simulink model "pid_azimuth"  (Simulink 5.0)
settings: Solver=ode5  StartTime=0.0  StopTime=30  FixedStep=.01  RelTol=1e-3
undefined symbols (not defined in the file): a, b, c, control_a, force_a, rpm_a
settings Model: LastModifiedBy=Administrator

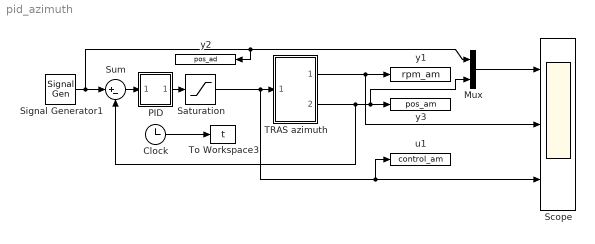
== system pid_azimuth ==
  Clock : Clock
  Mux : Mux  Inputs=2
  "PID " : Subsystem  AncestorBlock=|  mask(PID(2) Controller){P=a, I=b, D=c, N=100, S=1}
      | simulink_extras/Additional
      | Linear/PID Controller
      | (with Approximate
      | Derivative)
      mask prompts: P "Proportional:"; I "Integral:"; D "Derivative:"; N "Derivative divisor(N):"; S "Integral saturation(0-1)"
      mask help:
      | Enter Proportional(P), Integral(I), and Derivative(D) and divisor (N) terms.
      | P+I/s+Ds/(1/Ns+1)
      mask Help: This block implements a PID controller where parameters are entered for the Proportional, Integral and Derivative and divisor terms. Unmask this block to see how it works. The derivative term is implemented using an s/(s/N +1)  transfer function block. Making N large can create a "stiff" system.
      mask Display: disp('PID')
  Saturation : Saturate
  Scope : Scope  NumInputPorts=3
      settings: YMin=-5~-5~-5  YMax=5~5~5
  Signal Generator1 : SignalGenerator  WaveForm=square  Frequency=.05
  Sum : Sum  Inputs=|+-  SaturateOnIntegerOverflow=on
  TRAS azimuth : Subsystem
  To Workspace3 : ToWorkspace  VariableName=t  SampleTime=-1  SaveFormat=Array
  u1 : ToWorkspace  VariableName=control_am  SampleTime=-1  SaveFormat=Array
  y1 : ToWorkspace  VariableName=rpm_am  SampleTime=-1  SaveFormat=Array
  y2 : ToWorkspace  VariableName=pos_ad  SampleTime=-1  SaveFormat=Array
  y3 : ToWorkspace  VariableName=pos_am  SampleTime=-1  SaveFormat=Array
  wires:
  TRAS azimuth/1(rpm_a) -> y1/1, Scope/2
  Clock/1 -> To Workspace3/1
  Signal Generator1/1 -> Sum/1, Mux/1, y2/1
  Sum/1 -> "PID "/1(In_1)
  "PID "/1(Out_1) -> Saturation/1
  Mux/1 -> Scope/1
  Saturation/1 -> TRAS azimuth/1("ctrl_a "), Scope/3, u1/1
  TRAS azimuth/2(pos_am) -> y3/1, Mux/2, Sum/2

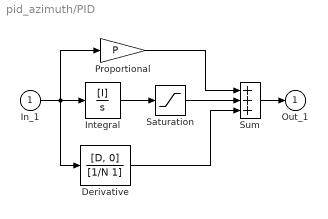
== system pid_azimuth/PID  ==
  In_1 : Inport
  Derivative : TransferFcn  Numerator=[D, 0]  Denominator=[1/N 1]
  Integral : TransferFcn  Numerator=[I]  Denominator=[1 0]
  Proportional : Gain  Gain=P  SaturateOnIntegerOverflow=on
  Saturation : Saturate  UpperLimit=S  LowerLimit=-S
  Sum : Sum  Inputs=+++  SaturateOnIntegerOverflow=on  InputSameDT=on
  Out_1 : Outport  InitialOutput=0
  wires:
  Sum/1 -> Out_1/1
  In_1/1 -> Derivative/1, Integral/1, Proportional/1
  Derivative/1 -> Sum/3
  Integral/1 -> Saturation/1
  Proportional/1 -> Sum/1
  Saturation/1 -> Sum/2

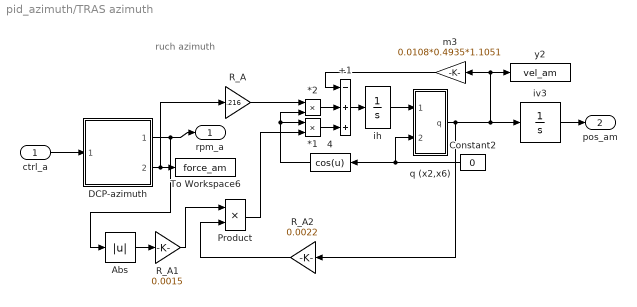
== system pid_azimuth/TRAS azimuth ==
  note: ruch azimuth
  "ctrl_a " : Inport
  *1 : Product  SaturateOnIntegerOverflow=on  InputSameDT=on
  *2 : Product  SaturateOnIntegerOverflow=on  InputSameDT=on
  +1 : Sum  Inputs=-++  SaturateOnIntegerOverflow=on  InputSameDT=on
  4 : Fcn  Orientation=left  Expr=cos(u)
  Abs : Abs  SaturateOnIntegerOverflow=on
  Constant2 : Constant  Orientation=left  Value=0
  DCP-azimuth : Subsystem
  Product : Product  SaturateOnIntegerOverflow=on  InputSameDT=on
  R_A : Gain  Gain=.216
  R_A1 : Gain  Gain=0.0015
  R_A2 : Gain  Orientation=left  Gain=0.0022
  To Workspace6 : ToWorkspace  VariableName=force_am  SampleTime=-1  SaveFormat=Array
  ih : Integrator
  iv3 : Integrator
  m3 : Gain  Orientation=left  Gain=0.0108*0.4935*1.1051
  q (x2,x6) : Subsystem
  y2 : ToWorkspace  VariableName=vel_am  SampleTime=-1  SaveFormat=Array
  rpm_a : Outport
  pos_am : Outport  Port=2
  wires:
  DCP-azimuth/2(FORCE_A) -> To Workspace6/1, R_A/1
  *1/1 -> +1/3
  m3/1 -> +1/1
  4/1 -> *1/1, *2/2
  *2/1 -> +1/2
  ih/1 -> q (x2,x6)/1(x2)
  q (x2,x6)/1(q) -> y2/1, m3/1, iv3/1, R_A2/1
  R_A/1 -> *2/1
  +1/1 -> ih/1
  Constant2/1 -> q (x2,x6)/2(x6), 4/1
  "ctrl_a "/1 -> DCP-azimuth/1(CTR_A)
  iv3/1 -> pos_am/1
  DCP-azimuth/1(RPM_A) -> rpm_a/1, Abs/1
  Product/1 -> *1/2
  R_A2/1 -> Product/2
  R_A1/1 -> Product/1
  Abs/1 -> R_A1/1

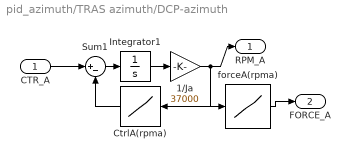
== system pid_azimuth/TRAS azimuth/DCP-azimuth ==
  CTR_A : Inport
  1/Ja : Gain  Gain=37000  ShowAdditionalParam=on  SaturateOnIntegerOverflow=on
  CtrlA(rpma) : Lookup  Orientation=left  InputValues=rpm_a  OutputValues=control_a  SaturateOnIntegerOverflow=on
  Integrator1 : Integrator
  Sum1 : Sum  Inputs=|+-  SaturateOnIntegerOverflow=on  InputSameDT=on
  forceA(rpma) : Lookup  InputValues=rpm_a  OutputValues=force_a  SaturateOnIntegerOverflow=on
  RPM_A : Outport
  FORCE_A : Outport  Port=2
  wires:
  Sum1/1 -> Integrator1/1
  CtrlA(rpma)/1 -> Sum1/2
  Integrator1/1 -> 1/Ja/1
  1/Ja/1 -> CtrlA(rpma)/1, forceA(rpma)/1, RPM_A/1
  CTR_A/1 -> Sum1/1
  forceA(rpma)/1 -> FORCE_A/1

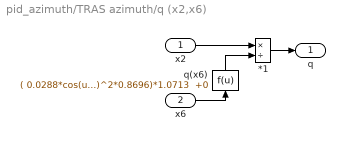
== system pid_azimuth/TRAS azimuth/q (x2,x6) ==
  x2 : Inport
  x6 : Inport  Port=2
  " q(x6)" : Fcn  Orientation=up  Expr="( 0.0288*cos(u)^2*0.8696)*1.0713  +0"
  *1 : Product  Inputs=*/  SaturateOnIntegerOverflow=on  InputSameDT=on
  q : Outport
  wires:
  *1/1 -> q/1
  x2/1 -> *1/1
  x6/1 -> " q(x6)"/1
  " q(x6)"/1 -> *1/2
